simulink model "CtrlStrct_CAN_Variant"  (R2018a)
settings: Solver=VariableStepAuto  StartTime=0.0  StopTime=10.0  FixedStep=sampletime  RelTol=1e-3  EnableMultiTasking=on
PreLoadFcn:
  | CtrlStrct_SmplCAN_BusInfo
undefined symbols (not defined in the file or in its folder): canChannel
libraries: canmsglib x106, canlib x35, simulink x1
(part 8 of 8)

== system CtrlStrct_CAN_Variant/CAN_Variant/VNT_Level_2_CAN/Steer_Ctrl/SteerCtrl_VehCAN_Rx/SteerCtrl_VehCAN_Receive50ms ==
  VehCAN_Msg : Inport
  function : TriggerPort  TriggerType=function-call  VariantControl=Variant
  Signal Specification : SignalSpecification
  SteerCtrl_VehCAN Unpack : canmsglib/CAN Unpack  CANdbFile=HEV_CANDB.dbc  MsgList=BrakeCtrl_VehCAN_Tx  MsgName=BrakeCtrl_VehCAN_Tx  MsgIDType=Extended (29-bit identifier)  MsgIdentifier=218062859  MsgLength=8  SignalInfo=BrkCtrl_Regen_brake_torque_reque$16$16$1$1$1$0$1.000000e-02$0$-300$300$#BrkCtrl_Vehicle_speed$0$16$1$2$1$0$1.000000e-01$0$0$180$#  NSignals=2  IDPort=off  TimestampPort=off  ErrorPort=off  RemotePort=off  LengthPort=off  StatusPort=off  StartBits=str2num('[int32(16);int32(0)]')  SignalSizes=str2num('[int32(16);int32(16)]')  ByteOrders=str2num('[int32(1);int32(1)]')  DataTypes=str2num('[int32(1);int32(2)]')  MultiplexTypes=str2num('[int32(1);int32(1)]')  MultiplexValues=str2num('[double(0);double(0)]')  Factors=str2num('[double(1.000000e-02);double(1.000000e-01)]')  Offsets=str2num('[double(0);double(0)]')  Minimums=str2num('[double(-300);double(0)]')  Maximums=str2num('[double(300);double(180)]')  ApplyMinMax=off
      settings: AttributesFormatString=<CANdbFile = %<CANdbFile>>  SourceProductName=Simulink Real-Time  SourceProductBaseCode=XP  DataFormat=CANdb specified signals
  Terminator4 : Terminator
  BrkCtrl_Vehicle_speed : Outport
  wires:
  SteerCtrl_VehCAN Unpack/1 -> Terminator4/1  "VehCAN_BrkCtrl_Regen_brake_torque_request"
  VehCAN_Msg/1 -> SteerCtrl_VehCAN Unpack/1
  SteerCtrl_VehCAN Unpack/2 -> Signal Specification/1  "VehCAN_BrkCtrl_Vehicle_speed"
  Signal Specification/1 -> BrkCtrl_Vehicle_speed/1  "BrkCtrl_Vehicle_speed"

== system CtrlStrct_CAN_Variant/CAN_Variant/VNT_Level_2_CAN/Transms_Ctrl/TransmCtrl_PwtrCAN_Rx/TransmCtrl_PwtrCAN_Receive_10ms ==
  PwtrCAN_Msg : Inport
  function : TriggerPort  TriggerType=function-call  VariantControl=Variant
  Signal Specification : SignalSpecification
  Signal Specification1 : SignalSpecification
  Terminator{1..3,5..9} (8 alike) : Terminator
  TransmCtrl_PwtrCAN Unpack : canmsglib/CAN Unpack  CANdbFile=HEV_CANDB.dbc  MsgList=Gateway_PwtrCAN_Tx_2  MsgName=Gateway_PwtrCAN_Tx_2  MsgIDType=Extended (29-bit identifier)  MsgIdentifier=218088325  MsgLength=8  SignalInfo=BdyCtrl_Door_open_flag_G$60$1$1$2$1$0$1$0$0$1$#BdyCtrl_Engine_hood_open_flg_G$59$1$1$2$1$0$1$0$0$1$#BdyCtrl_Idlestop_cancel_G$58$1$1$2$1$0$1$0$0$1$#BrkCtrl_Regen_brake_torque_re_G$16$16$1$1$1$0$1.000000e-02$0$-300$300$#BrkCtrl_Vehicle_speed_G$0$16$1$2$1$0$1.000000e-01$0$0$180$#HVAC_Ctrl_Idlestop_cancel_G$57$1$1$2$1$0$1$0$0$1$#HVAC_Ctrl_Idlestop_enbl_G$56$1$1$2$1$0$1$0$0$1$#StrgCtrl_Steer_angle_G$32$16$1$1$1$0$3.125000e-02$0$-720$720$#  NSignals=8  IDPort=off  TimestampPort=off  ErrorPort=off  RemotePort=off  LengthPort=off  StatusPort=off  StartBits=str2num('[int32(60);int32(59);int32(58);int32(16);int32(0);int32(57);int32(56);int32(32)]')  SignalSizes=str2num('[int32(1);int32(1);int32(1);int32(16);int32(16);int32(1);int32(1);int32(16)]')  ByteOrders=str2num('[int32(1);int32(1);int32(1);int32(1);int32(1);int32(1);int32(1);int32(1)]')  DataTypes=str2num('[int32(2);int32(2);int32(2);int32(1);int32(2);int32(2);int32(2);int32(1)]')  MultiplexTypes=str2num('[int32(1);int32(1);int32(1);int32(1);int32(1);int32(1);int32(1);int32(1)]')  MultiplexValues=str2num('[double(0);double(0);double(0);double(0);double(0);double(0);double(0);double(0)]')  Factors=str2num('[double(1);double(1);double(1);double(1.000000e-02);double(1.000000e-01);double(1);double(1);double(3.125000e-02)]')  Offsets=str2num('[double(0);double(0);double(0);double(0);double(0);double(0);double(0);double(0)]')  Minimums=str2num('[double(0);double(0);double(0);double(-300);double(0);double(0);double(0);double(-720)]')  Maximums=str2num('[double(1);double(1);double(1);double(300);double(180);double(1);double(1);double(720)]')  ApplyMinMax=off
      settings: AttributesFormatString=<CANdbFile = %<CANdbFile>>  SourceProductName=Simulink Real-Time  SourceProductBaseCode=XP  DataFormat=CANdb specified signals
  TransmCtrl_PwtrCAN Unpack2 : canmsglib/CAN Unpack  CANdbFile=HEV_CANDB.dbc  MsgList=EngineCtrl_PwtrCAN_Tx  MsgName=EngineCtrl_PwtrCAN_Tx  MsgIDType=Extended (29-bit identifier)  MsgIdentifier=218050560  MsgLength=8  SignalInfo=EngCtrl_Engine_speed$0$16$1$2$1$0$1.250000e-01$0$0$8192$#EngCtrl_Engine_torque_actual$16$16$1$1$1$0$1.562500e-02$0$-300$300$#  NSignals=2  IDPort=off  TimestampPort=off  ErrorPort=off  RemotePort=off  LengthPort=off  StatusPort=off  StartBits=str2num('[int32(0);int32(16)]')  SignalSizes=str2num('[int32(16);int32(16)]')  ByteOrders=str2num('[int32(1);int32(1)]')  DataTypes=str2num('[int32(2);int32(1)]')  MultiplexTypes=str2num('[int32(1);int32(1)]')  MultiplexValues=str2num('[double(0);double(0)]')  Factors=str2num('[double(1.250000e-01);double(1.562500e-02)]')  Offsets=str2num('[double(0);double(0)]')  Minimums=str2num('[double(0);double(-300)]')  Maximums=str2num('[double(8192);double(300)]')  ApplyMinMax=off
      settings: AttributesFormatString=<CANdbFile = %<CANdbFile>>  SourceProductName=Simulink Real-Time  SourceProductBaseCode=XP  DataFormat=CANdb specified signals
  BrkCtrl_Vehicle_speed : Outport
  EngCtrl_Engine_speed : Outport  Port=2
  wires:
  TransmCtrl_PwtrCAN Unpack/2 -> Terminator5/1
  TransmCtrl_PwtrCAN Unpack/8 -> Terminator9/1
  TransmCtrl_PwtrCAN Unpack/4 -> Terminator3/1
  TransmCtrl_PwtrCAN Unpack/7 -> Terminator8/1
  TransmCtrl_PwtrCAN Unpack/6 -> Terminator7/1
  TransmCtrl_PwtrCAN Unpack/3 -> Terminator6/1
  TransmCtrl_PwtrCAN Unpack/1 -> Terminator1/1
  TransmCtrl_PwtrCAN Unpack2/2 -> Terminator2/1  "PwtrCAN_EngCtrl_Engine_torque_actual"
  PwtrCAN_Msg/1 -> TransmCtrl_PwtrCAN Unpack2/1, TransmCtrl_PwtrCAN Unpack/1
  TransmCtrl_PwtrCAN Unpack/5 -> Signal Specification/1  "PwtrCAN_BrkCtrl_Vehicle_speed"
  TransmCtrl_PwtrCAN Unpack2/1 -> Signal Specification1/1  "PwtrCAN_EngCtrl_Engine_speed"
  Signal Specification/1 -> BrkCtrl_Vehicle_speed/1  "BrkCtrl_Vehicle_speed"
  Signal Specification1/1 -> EngCtrl_Engine_speed/1  "EngCtrl_Engine_speed"

== system CtrlStrct_CAN_Variant/CAN_Variant/VNT_Level_2_CAN/VM_Ctrl/VM_Ctrl_VehCAN_Rx/VM_Ctrl_VehCAN_Receive_50ms ==
  VehCAN_Msg : Inport
  function : TriggerPort  TriggerType=function-call  VariantControl=Variant
  Signal Specification : SignalSpecification
  Terminator4 : Terminator
  VM_Ctrl_VehCAN Unpack : canmsglib/CAN Unpack  CANdbFile=HEV_CANDB.dbc  MsgList=BrakeCtrl_VehCAN_Tx  MsgName=BrakeCtrl_VehCAN_Tx  MsgIDType=Extended (29-bit identifier)  MsgIdentifier=218062859  MsgLength=8  SignalInfo=BrkCtrl_Regen_brake_torque_reque$16$16$1$1$1$0$1.000000e-02$0$-300$300$#BrkCtrl_Vehicle_speed$0$16$1$2$1$0$1.000000e-01$0$0$180$#  NSignals=2  IDPort=off  TimestampPort=off  ErrorPort=off  RemotePort=off  LengthPort=off  StatusPort=off  StartBits=str2num('[int32(16);int32(0)]')  SignalSizes=str2num('[int32(16);int32(16)]')  ByteOrders=str2num('[int32(1);int32(1)]')  DataTypes=str2num('[int32(1);int32(2)]')  MultiplexTypes=str2num('[int32(1);int32(1)]')  MultiplexValues=str2num('[double(0);double(0)]')  Factors=str2num('[double(1.000000e-02);double(1.000000e-01)]')  Offsets=str2num('[double(0);double(0)]')  Minimums=str2num('[double(-300);double(0)]')  Maximums=str2num('[double(300);double(180)]')  ApplyMinMax=off
      settings: AttributesFormatString=<CANdbFile = %<CANdbFile>>  SourceProductName=Simulink Real-Time  SourceProductBaseCode=XP  DataFormat=CANdb specified signals
  BrkCtrl_Vehicle_speed : Outport
  wires:
  VM_Ctrl_VehCAN Unpack/2 -> Signal Specification/1  "VehCAN_BrkCtrl_Vehicle_speed"
  VM_Ctrl_VehCAN Unpack/1 -> Terminator4/1  "VehCAN_BrkCtrl_Regen_brake_torque_request"
  VehCAN_Msg/1 -> VM_Ctrl_VehCAN Unpack/1
  Signal Specification/1 -> BrkCtrl_Vehicle_speed/1  "BrkCtrl_Vehicle_speed"
